simulink subsystem "Battery"  (R2022b)
settings: Solver=VariableStepAuto  StartTime=0.0  StopTime=10.0  RelTol=1e-3
undefined symbols (not defined in the file): batt_cap_init, OCV, OCV_SoC, PlntBattNumCellPar, PlntBattNumCellSer, soc_init
libraries: autolibdatasheetbattery x1
settings Model: ModifiedByFormat=The MathWorks, Inc.  Creator=The MathWorks, Inc.  LastModifiedBy=The MathWorks, Inc.
settings SolverCC: MaxZcPerStep=1
settings DebuggingCC: UnconnectedInputMsg=warning  UnconnectedOutputMsg=warning  UnconnectedLineMsg=warning
settings ModelReferenceCC: EnableRefExpFcnMdlSchedulingChecks=on
settings RTWCC: DLArmComputeVersion=19.05

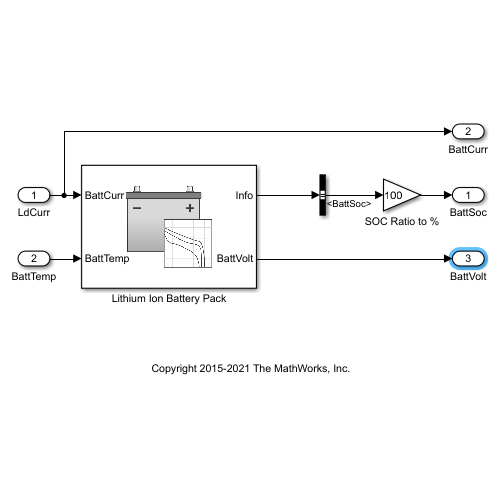
[thumbnail: Simulink's stored preview of the top-level diagram]
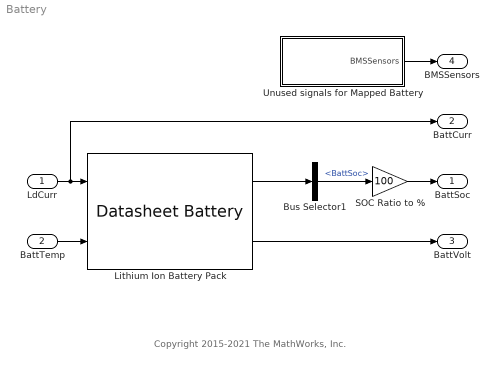
== system Battery ==
  note: Copyright 2015-2021 The MathWorks, Inc.
  LdCurr : Inport
  BattTemp : Inport  Port=2
  Bus Selector1 : BusSelector  OutputSignals=BattSoc
  Lithium Ion Battery Pack : autolibdatasheetbattery/Datasheet Battery  CapacityCtrl=Parameter  OutputVlt=Filtered  BattChargeMax=(batt_cap_init/soc_init)/PlntBattNumCellPar  Em=OCV/PlntBattNumCellSer  CapLUTBp=OCV_SoC/100  RInt=PlntBattIntrnRes  BattTempBp=PlntBattTempBpt  CapSOCBp=PlntBattSocBpt  Ns=PlntBattNumCellSer  Np=PlntBattNumCellPar  BattCapInit=batt_cap_init/PlntBattNumCellPar  Tc=PlntBattTimeCnst  Vinit=interp1(OCV_SoC/100, OCV, soc_init)  RefBlkName='autolibdatasheetbattery/Datasheet Battery'
  SOC Ratio to % : Gain  Gain=100
  Unused signals for Mapped Battery : Subsystem
  BattSoc : Outport  VectorParamsAs1DForOutWhenUnconnected=off
  BattCurr : Outport  Port=2  VectorParamsAs1DForOutWhenUnconnected=off
  BattVolt : Outport  Port=3  VectorParamsAs1DForOutWhenUnconnected=off
  BMSSensors : Outport  Port=4  VectorParamsAs1DForOutWhenUnconnected=off
  wires:
  Unused signals for Mapped Battery/1(BMSSensors) -> BMSSensors/1
  Lithium Ion Battery Pack/1 -> Bus Selector1/1
  SOC Ratio to %/1 -> BattSoc/1
  LdCurr/1 -> Lithium Ion Battery Pack/1, BattCurr/1
  Bus Selector1/1 -> SOC Ratio to %/1  "<BattSoc>"
  BattTemp/1 -> Lithium Ion Battery Pack/2
  Lithium Ion Battery Pack/2 -> BattVolt/1

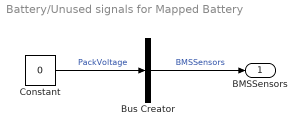
== system Battery/Unused signals for Mapped Battery ==
  Bus Creator : BusCreator  Inputs=1
  Constant : Constant  Value=0  SampleTime=-1
  BMSSensors : Outport
  wires:
  Bus Creator/1 -> BMSSensors/1  "BMSSensors"
  Constant/1 -> Bus Creator/1  "PackVoltage"
